simulink model "pendulum_model"  (R2025b)
settings: Solver=ode4  StartTime=0.0  StopTime=SIM_TIME  FixedStep=STEP_SIZE  RelTol=1e-3
values from neighbouring files (symbols this model uses):
  b = 0    [params.m]
  c = 0    [params.m]
  c_belt = 2*zeta*sqrt(Meff*k_belt)    [params.m]
  CURRENT_QUANTIZATION = ADC_QUANTIZATION*1/VOLT_PER_AMP    (= 0.002685546875)    [params.m]
  CURRENT_SATURATION = MID_REF/VOLT_PER_AMP    (= 5.5)    [params.m]
  d = 0    [params.m]
  g = 9.82    [params.m]
  I = (1/3) * m * l^2    (= 0.00210444819888)    [params.m]
  i0 = 0    [pendulum_sim.m]
  J = 115*1e-7    (= 1.15e-05)    [params.m]
  k_belt = 1e3    (= 1000)    [params.m]
  K_lqr = zeros(1,7)    [pendulum_sim.m]
  Ke = Kt    (= 0.0797)    [params.m]
  Kt = 79.7e-3    (= 0.0797)    [params.m]
  L = 708e-6    (= 0.000708)    [params.m]
  l = Ltotal/2    (= 0.2)    [params.m]
  m = 7850*Ltotal*(4e-3)^2*pi    (= 0.157833614916)    [params.m]
  M = 54e-3    (= 0.054)    [params.m]
  Mr = 6.5e-3    (= 0.0065)    [params.m]
  phi_dot0 = 0    [pendulum_sim.m]
  r = PULLEY_D/2    (= 0.00636619772368)    [params.m]
  R = 2.59    [params.m]    (also in pendulum_sim.m = 0.01)
  SIM_IDEAL_MEASUREMENT = 1    [pendulum_sim.m]
  SIM_OPEN_LOOP = 0    [pendulum_sim.m]
  STEP_CTRL = 1e-3    (= 0.001)    [params.m]
  theta0 = pi - deg2rad(3)    [pendulum_sim.m]
  theta_dot0 = 0    [pendulum_sim.m]
  VOLTAGE_SATURATION = 12    [params.m]
  x0 = 0    [pendulum_sim.m]
  x_dot0 = 0    [pendulum_sim.m]
settings Model: Creator=farfar  LastModifiedBy=farfar
settings DataIOCC: ReturnWorkspaceOutputs=off  OutputSaveName=tsim

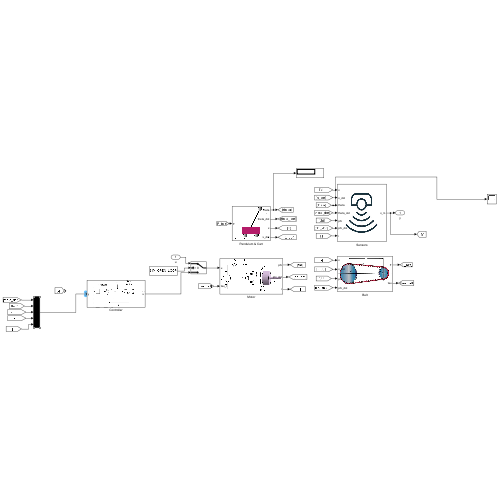
[thumbnail: Simulink's stored preview of the top-level diagram]
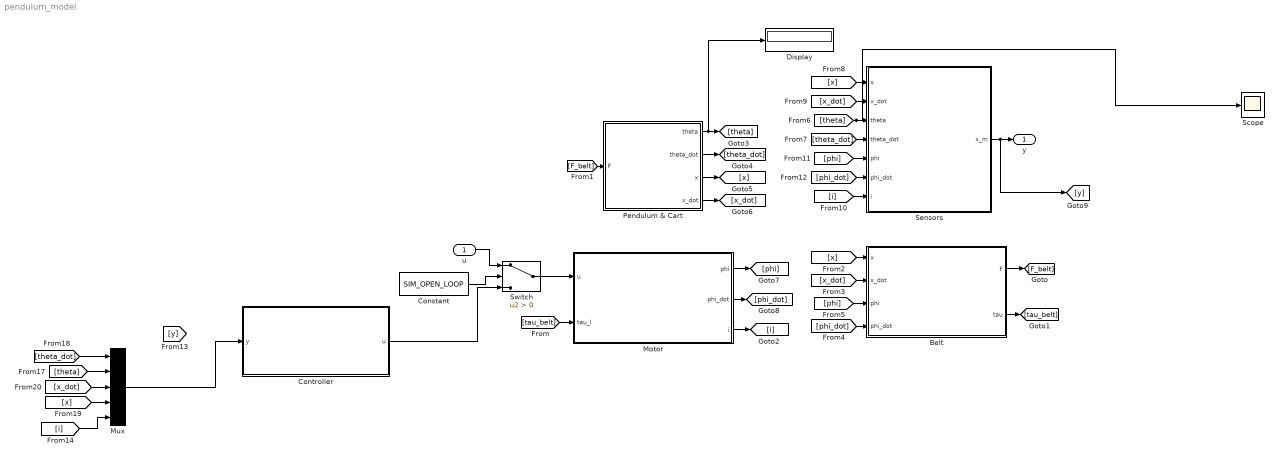
== system pendulum_model ==
  u : Inport
  Belt : Subsystem
      mask Display: image('belt_block_cover.png');
  Constant : Constant  Value=SIM_OPEN_LOOP
  Controller : Subsystem
      mask Display: image('controller_block_cover.png');
  Display : Display
  Motor : Subsystem
      mask Display: image('motor_block_cover.png');
  Mux : Mux  Inputs=5
  Pendulum & Cart : Subsystem
      mask Display: image('pendulum_block_cover.png');
  Scope : Scope
      settings: ActiveDisplayYMinimum=-34.3946088054704  ActiveDisplayYMaximum=56.783561052906329
  Sensors : Subsystem
      mask Display: image('sensor_block_cover.png');
  Switch : Switch  Criteria=u2 > Threshold  SaturateOnIntegerOverflow=off  InputSameDT=off
  y : Outport
  wires:
  Pendulum & Cart/1(theta) -> Display/1, [theta]
  Pendulum & Cart/2(theta_dot) -> [theta_dot]
  Constant/1 -> Switch/2
  Switch/1 -> Motor/1(u)
  u/1 -> Switch/1
  Belt/2(tau) -> [tau_belt]
  Belt/1(F) -> [F_belt]
  [tau_belt] -> Motor/2(tau_l)
  [F_belt] -> Pendulum & Cart/1(F)
  Motor/3(i) -> [i]
  Pendulum & Cart/4(x_dot) -> [x_dot]
  Pendulum & Cart/3(x) -> [x]
  Motor/2(phi_dot) -> [phi_dot]
  Motor/1(phi) -> [phi]
  [x] -> Belt/1(x)
  [x_dot] -> Belt/2(x_dot)
  [phi_dot] -> Belt/4(phi_dot)
  [phi] -> Belt/3(phi)
  [i] -> Sensors/7(i)
  [theta_dot] -> Sensors/4(theta_dot)
  [theta] -> Scope/1, Sensors/3(theta)
  [x_dot] -> Sensors/2(x_dot)
  [x] -> Sensors/1(x)
  [phi] -> Sensors/5(phi)
  [phi_dot] -> Sensors/6(phi_dot)
  Controller/1(u) -> Switch/3
  Sensors/1(x_m) -> [y], y/1
  [i] -> Mux/5
  [x_dot] -> Mux/3
  [x] -> Mux/4
  [theta] -> Mux/2
  [theta_dot] -> Mux/1
  Mux/1 -> Controller/1(y)

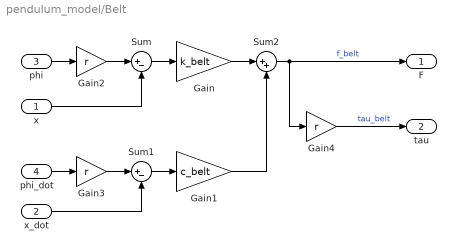
== system pendulum_model/Belt ==
  x : Inport
  x_dot : Inport  Port=2
  phi : Inport  Port=3
  phi_dot : Inport  Port=4
  Gain : Gain  Gain=k_belt
  Gain1 : Gain  Gain=c_belt
  Gain2 : Gain  Gain=r
  Gain3 : Gain  Gain=r
  Gain4 : Gain  Gain=r
  Sum : Sum  Inputs=|+-
  Sum1 : Sum  Inputs=|+-
  Sum2 : Sum  Inputs=|++
  F : Outport
  tau : Outport  Port=2
  wires:
  Sum1/1 -> Gain1/1
  Sum/1 -> Gain/1
  phi/1 -> Gain2/1
  phi_dot/1 -> Gain3/1
  Gain2/1 -> Sum/1
  Gain3/1 -> Sum1/1
  x/1 -> Sum/2
  x_dot/1 -> Sum1/2
  Sum2/1 -> Gain4/1, F/1  "f_belt"
  Gain/1 -> Sum2/1
  Gain1/1 -> Sum2/2
  Gain4/1 -> tau/1  "tau_belt"

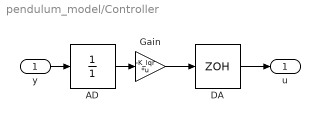
== system pendulum_model/Controller ==
  y : Inport
  AD : DiscreteTransferFcn  Denominator=[1]  SampleTime=STEP_CTRL
  DA : ZeroOrderHold  SampleTime=STEP_CTRL
  Gain : Gain  Gain=-K_lqr  Multiplication=Matrix(K*u) (u vector)
  u : Outport
  wires:
  y/1 -> AD/1
  Gain/1 -> DA/1
  DA/1 -> u/1
  AD/1 -> Gain/1

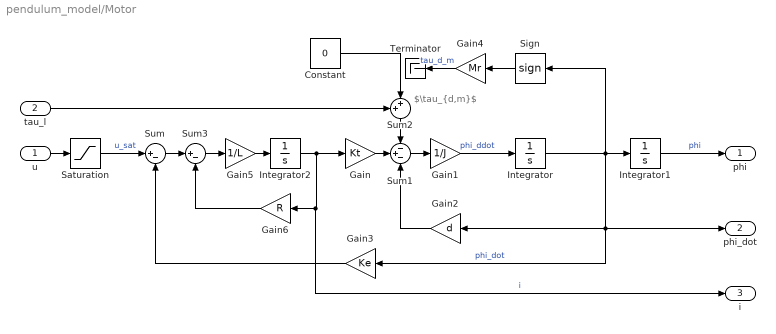
== system pendulum_model/Motor ==
  note: $\tau_{d,m}$
  u : Inport
  tau_l : Inport  Port=2
  Constant : Constant  Value=0
  Gain : Gain  Gain=Kt
  Gain1 : Gain  Gain=1/J
  Gain2 : Gain  Gain=d
  Gain3 : Gain  Gain=Ke
  Gain4 : Gain  Gain=Mr
  Gain5 : Gain  Gain=1/L
  Gain6 : Gain  Gain=R
  Integrator : Integrator  Priority=5  InitialCondition=phi_dot0  ContinuousStateAttributes='motor.angular.velocity'
  Integrator1 : Integrator  Tag=6  ContinuousStateAttributes='motor.angular.position'
  Integrator2 : Integrator  Priority=7  InitialCondition=i0  ContinuousStateAttributes='motor.current'
  Saturation : Saturate  UpperLimit=VOLTAGE_SATURATION  LowerLimit=-VOLTAGE_SATURATION
  Sign : Signum  ZeroCross=off
  Sum : Sum  Inputs=|+-
  Sum1 : Sum  Inputs=-+-
  Sum2 : Sum  Inputs=++|
  Sum3 : Sum  Inputs=|+-
  Terminator : Terminator
  phi : Outport
  phi_dot : Outport  Port=2
  i : Outport  Port=3
  wires:
  Gain2/1 -> Sum1/3
  Gain1/1 -> Integrator/1  "phi_ddot"
  Sum/1 -> Sum3/1
  Gain3/1 -> Sum/2
  Gain4/1 -> Terminator/1  "tau_d_m"
  Sign/1 -> Gain4/1
  Gain/1 -> Sum1/2
  Integrator/1 -> Sign/1, Gain2/1, Gain3/1, phi_dot/1, Integrator1/1  "phi_dot"
  Sum1/1 -> Gain1/1
  Sum2/1 -> Sum1/1
  tau_l/1 -> Sum2/1
  Integrator1/1 -> phi/1  "phi"
  u/1 -> Saturation/1
  Integrator2/1 -> i/1, Gain6/1, Gain/1  "i"
  Gain5/1 -> Integrator2/1
  Sum3/1 -> Gain5/1
  Gain6/1 -> Sum3/2
  Saturation/1 -> Sum/1  "u_sat"
  Constant/1 -> Sum2/2

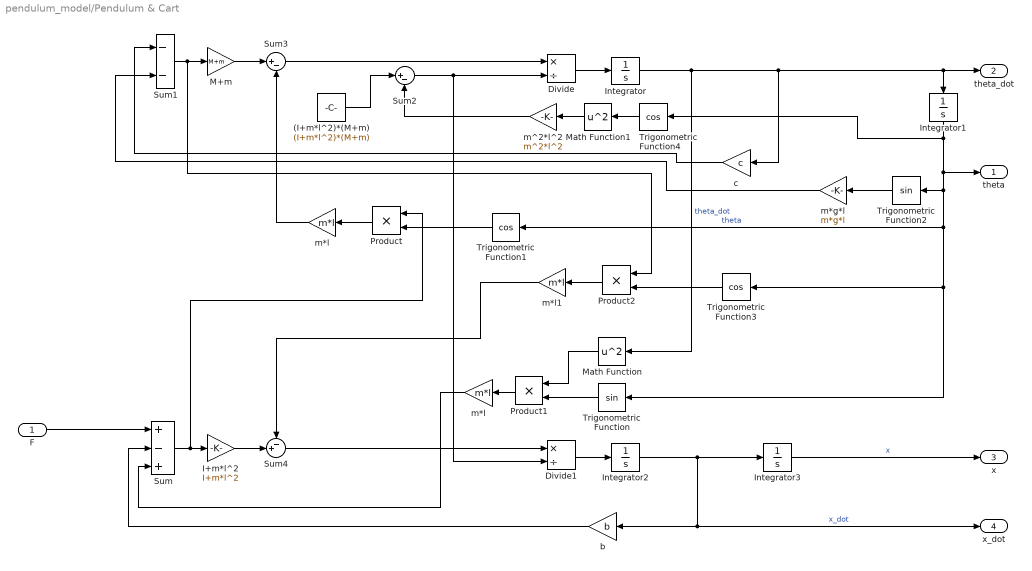
== system pendulum_model/Pendulum & Cart ==
  F : Inport
  (I+m*l^2)*(M+m) : Constant  Value=(I+m*l^2)*(M+m)
  Divide : Product  Inputs=*/
  Divide1 : Product  Inputs=*/
  I+m*l^2 : Gain  Gain=I+m*l^2
  Integrator : Integrator  Priority=1  InitialCondition=theta_dot0  ContinuousStateAttributes='pendulum.angular.velocity'
  Integrator1 : Integrator  Priority=2  InitialCondition=theta0  UpperSaturationLimit=pi  LowerSaturationLimit=-pi  ContinuousStateAttributes='pendulum.angular.position'
  Integrator2 : Integrator  Priority=3  InitialCondition=x_dot0  ContinuousStateAttributes='trolley.horizontal.velocity'
  Integrator3 : Integrator  Priority=4  InitialCondition=x0  ContinuousStateAttributes='trolley.horizontal.position'
  M+m : Gain  Gain=M+m
  Math Function : Math  Operator=square
  Math Function1 : Math  Operator=square
  Product : Product
  Product1 : Product
  Product2 : Product
  Sum : Sum  Inputs=+-+
  Sum1 : Sum  Inputs=--
  Sum2 : Sum  Inputs=|+-
  Sum3 : Sum  Inputs=|+-
  Sum4 : Sum  Inputs=-+|
  Trigonometric Function : Trigonometry
  Trigonometric Function1 : Trigonometry  Operator=cos
  Trigonometric Function2 : Trigonometry
  Trigonometric Function3 : Trigonometry  Operator=cos
  Trigonometric Function4 : Trigonometry  Operator=cos
  b : Gain  Gain=b
  c : Gain  Gain=c
  m*g*l : Gain  Gain=m*g*l
  m*l : Gain  Gain=m*l
  "m*l " : Gain  Gain=m*l
  m*l1 : Gain  Gain=m*l
  m^2*l^2 : Gain  Gain=m^2*l^2
  theta : Outport
  theta_dot : Outport  Port=2
  x : Outport  Port=3
  x_dot : Outport  Port=4
  wires:
  m^2*l^2/1 -> Sum2/2
  Product/1 -> m*l/1
  F/1 -> Sum/1
  Sum3/1 -> Divide/1
  M+m/1 -> Sum3/1
  I+m*l^2/1 -> Sum4/2
  Integrator2/1 -> x_dot/1, b/1, Integrator3/1  "x_dot"
  Divide/1 -> Integrator/1
  m*g*l/1 -> Sum1/2
  Sum1/1 -> Product2/1, M+m/1
  Divide1/1 -> Integrator2/1
  Integrator3/1 -> x/1  "x"
  Math Function/1 -> Product1/1
  Trigonometric Function3/1 -> Product2/2
  Trigonometric Function/1 -> Product1/2
  Integrator1/1 -> Trigonometric Function/1, Trigonometric Function3/1, Trigonometric Function1/1, Trigonometric Function2/1, theta/1, Trigonometric Function4/1  "theta"
  Product2/1 -> m*l1/1
  b/1 -> Sum/2
  Math Function1/1 -> m^2*l^2/1
  Sum2/1 -> Divide1/2, Divide/2
  Trigonometric Function4/1 -> Math Function1/1
  m*l/1 -> Sum3/2
  Trigonometric Function1/1 -> Product/2
  "m*l "/1 -> Sum/3
  Product1/1 -> "m*l "/1
  m*l1/1 -> Sum4/1
  Integrator/1 -> Math Function/1, c/1, Integrator1/1, theta_dot/1  "theta_dot"
  (I+m*l^2)*(M+m)/1 -> Sum2/1
  Trigonometric Function2/1 -> m*g*l/1
  c/1 -> Sum1/1
  Sum/1 -> Product/1, I+m*l^2/1
  Sum4/1 -> Divide1/1

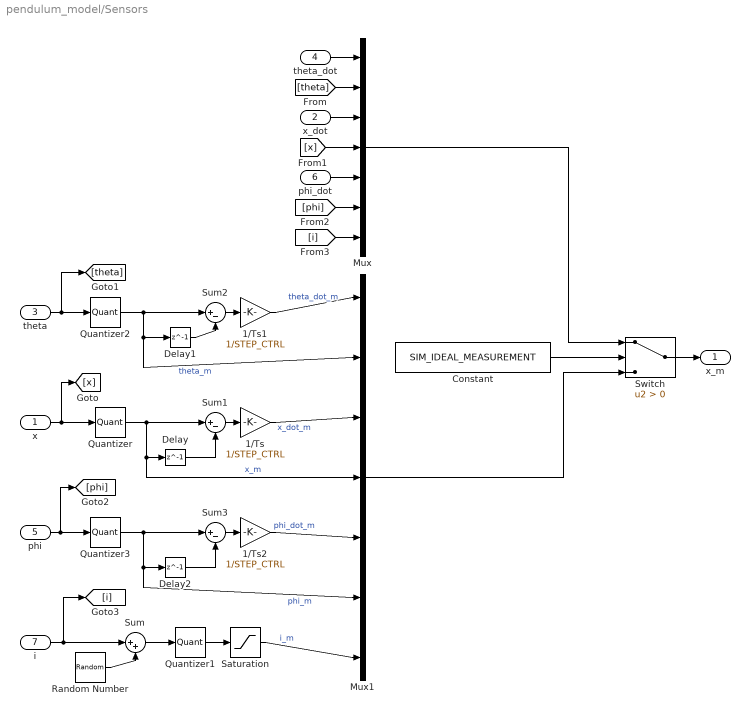
== system pendulum_model/Sensors ==
  x : Inport
  x_dot : Inport  Port=2
  theta : Inport  Port=3
  theta_dot : Inport  Port=4
  phi : Inport  Port=5
  phi_dot : Inport  Port=6
  i : Inport  Port=7
  1/Ts : Gain  Gain=1/STEP_CTRL
  1/Ts1 : Gain  Gain=1/STEP_CTRL
  1/Ts2 : Gain  Gain=1/STEP_CTRL
  Constant : Constant  Value=SIM_IDEAL_MEASUREMENT
  Delay : Delay  DelayLength=1  SampleTime=STEP_CTRL
  Delay1 : Delay  DelayLength=1  SampleTime=STEP_CTRL
  Delay2 : Delay  DelayLength=1  SampleTime=STEP_CTRL
  Mux : Mux  Inputs=7
  Mux1 : Mux  Inputs=7
  Quantizer : Quantizer  QuantizationInterval=LINEAR_QUANTIZATION
  Quantizer1 : Quantizer  QuantizationInterval=CURRENT_QUANTIZATION
  Quantizer2 : Quantizer  QuantizationInterval=ANGULAR_QUANTIZATION
  Quantizer3 : Quantizer  QuantizationInterval=ANGULAR_QUANTIZATION
  Random Number : RandomNumber  Variance=CURRENT_QUANTIZATION*2  SampleTime=STEP_CTRL
  Saturation : Saturate  UpperLimit=CURRENT_SATURATION  LowerLimit=-CURRENT_SATURATION
  Sum : Sum  Inputs=|++
  Sum1 : Sum  Inputs=|+-
  Sum2 : Sum  Inputs=|+-
  Sum3 : Sum  Inputs=|+-
  Switch : Switch  Criteria=u2 > Threshold  SaturateOnIntegerOverflow=off  InputSameDT=off
  x_m : Outport
  wires:
  x/1 -> [x], Quantizer/1
  Random Number/1 -> Sum/2
  Sum/1 -> Quantizer1/1
  Quantizer1/1 -> Saturation/1
  i/1 -> [i], Sum/1
  Saturation/1 -> Mux1/7  "i_m"
  theta/1 -> [theta], Quantizer2/1
  phi/1 -> [phi], Quantizer3/1
  Sum1/1 -> 1/Ts/1
  Quantizer/1 -> Mux1/4, Delay/1, Sum1/1  "x_m"
  Delay/1 -> Sum1/2
  1/Ts/1 -> Mux1/3  "x_dot_m"
  Delay1/1 -> Sum2/2
  Quantizer2/1 -> Mux1/2, Delay1/1, Sum2/1  "theta_m"
  Sum2/1 -> 1/Ts1/1
  1/Ts1/1 -> Mux1/1  "theta_dot_m"
  Quantizer3/1 -> Mux1/6, Delay2/1, Sum3/1  "phi_m"
  Delay2/1 -> Sum3/2
  1/Ts2/1 -> Mux1/5  "phi_dot_m"
  Sum3/1 -> 1/Ts2/1
  Constant/1 -> Switch/2
  [theta] -> Mux/2
  theta_dot/1 -> Mux/1
  phi_dot/1 -> Mux/5
  [x] -> Mux/4
  [phi] -> Mux/6
  [i] -> Mux/7
  Mux/1 -> Switch/1
  Mux1/1 -> Switch/3
  x_dot/1 -> Mux/3
  Switch/1 -> x_m/1
